simulink model "test"  (Simulink 6.5)
settings: Solver=FixedStepDiscrete  StartTime=0.0  StopTime=10E16  FixedStep=1  RelTol=1e-3
settings Model: Creator=henrik  LastModifiedBy=research
settings OptimizationCC: BooleanDataType=off
settings DebuggingCC: SolverPrmCheckMsg=none  MultiTaskDSMMsg=warning  MultiTaskCondExecSysMsg=none  StrictBusMsg=None
settings HardwareCC: TargetUnknown=on
settings RTWCC: IncludeERTFirstTime=on

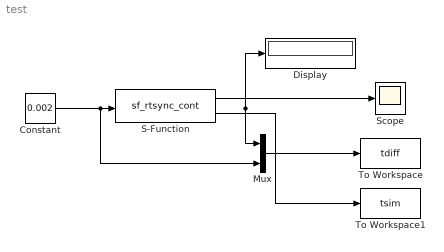
== system test ==
  Constant : Constant  Value=0.002  OutDataType=sfix(16)  ConRadixGroup=Use specified scaling  OutScaling=2^0  SampleTime=inf  FramePeriod=inf
  Display : Display
  Mux : Mux  Inputs=2
  S-Function : S-Function  FunctionName=sf_rtsync_cont  Parameters=1
  Scope : Scope
      settings: TimeRange=5000  YMin=-4.33681e-018  YMax=0.0575
  To Workspace : ToWorkspace  VariableName=tdiff  SampleTime=-1  SaveFormat=Array
  To Workspace1 : ToWorkspace  VariableName=tsim  SampleTime=-1  SaveFormat=Array
  wires:
  S-Function/1 -> Display/1, Mux/1, Scope/1
  Constant/1 -> S-Function/1, Mux/2
  Mux/1 -> To Workspace/1
  S-Function/2 -> To Workspace1/1
